simulink model "Vereinfachte_Dehtellersteuerung"  (R2021a)
settings: Solver=ode3  StartTime=0.0  StopTime=10  FixedStep=0.01  RelTol=1e-3
undefined symbols (not defined in the file): A, I, igetr, K, MRK, PHI, Ra, U
settings Model: Creator=Oceaner  LastModifiedBy=Oceaner

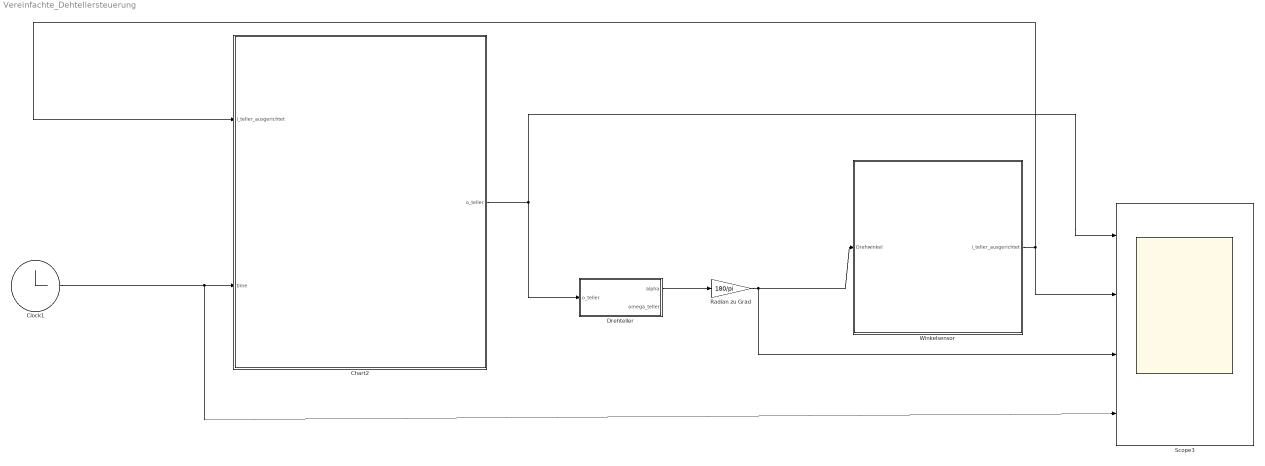
== system Vereinfachte_Dehtellersteuerung ==
  Chart2 : Stateflow chart  TreatAsAtomicUnit=on
  Clock1 : Clock
  Drehteller : Subsystem
  Radian zu Grad : Gain  Gain=180/pi
  Scope3 : Scope  NumInputPorts=4
  Winkelsensor : Stateflow chart  TreatAsAtomicUnit=on
  wires:
  Clock1/1 -> Scope3/4, Chart2/2(time)
  Winkelsensor/1(i_teller_ausgerichtet) -> Chart2/1(i_teller_ausgerichtet), Scope3/2
  Drehteller/1(alpha) -> Radian zu Grad/1
  Chart2/1(o_teller) -> Drehteller/1(o_teller), Scope3/1
  Radian zu Grad/1 -> Scope3/3, Winkelsensor/1(Drehwinkel)

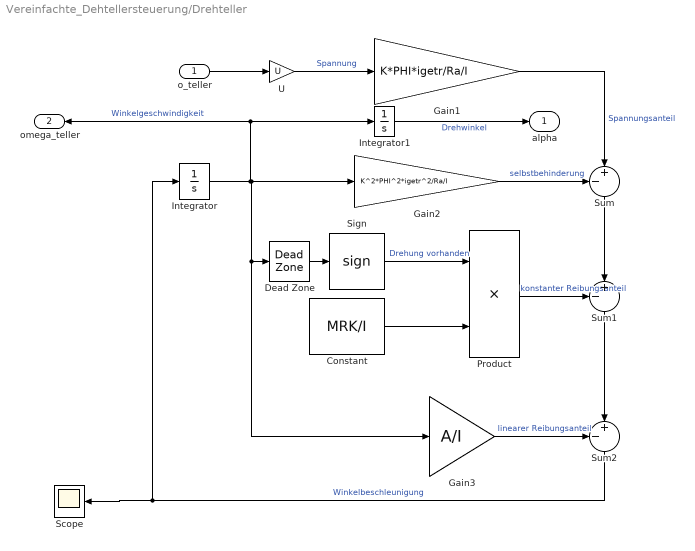
== system Vereinfachte_Dehtellersteuerung/Drehteller ==
  o_teller : Inport
  Constant : Constant  Value=MRK/I
  Dead Zone : DeadZone  SaturateOnIntegerOverflow=on
  Gain1 : Gain  Gain=K*PHI*igetr/Ra/I
  Gain2 : Gain  Gain=K^2*PHI^2*igetr^2/Ra/I
  Gain3 : Gain  Gain=A/I
  Integrator : Integrator
  Integrator1 : Integrator
  Product : Product
  Scope : Scope
  Sign : Signum
  Sum : Sum  Inputs=-+|
  Sum1 : Sum  Inputs=-+|
  Sum2 : Sum  Inputs=-+|
  U : Gain  Gain=U
  alpha : Outport
  omega_teller : Outport  Port=2
  wires:
  U/1 -> Gain1/1  "Spannung"
  Product/1 -> Sum1/1  "konstanter Reibungsanteil"
  Integrator/1 -> Gain2/1, Gain3/1, Dead Zone/1, omega_teller/1, Integrator1/1  "Winkelgeschwindigkeit"
  Gain1/1 -> Sum/2  "Spannungsanteil"
  Sum1/1 -> Sum2/2
  Sum/1 -> Sum1/2
  o_teller/1 -> U/1
  Gain2/1 -> Sum/1  "selbstbehinderung"
  Sign/1 -> Product/1  "Drehung vorhanden"
  Dead Zone/1 -> Sign/1
  Gain3/1 -> Sum2/1  "linearer Reibungsanteil"
  Sum2/1 -> Scope/1, Integrator/1  "Winkelbeschleunigung"
  Constant/1 -> Product/2
  Integrator1/1 -> alpha/1  "Drehwinkel"

== stateflow chart Vereinfachte_Dehtellersteuerung/Chart2 ==
  state pufferstate
  state beginnt
    en:o_teller=1;
  state aus
    en:o_teller=0;
  beginnt -> pufferstate : after(0.5,sec)
  pufferstate -> aus : [i_teller_ausgerichtet==1]
  (default) -> aus
  aus -> beginnt : after(2,sec)
  data: i_teller_ausgerichtet input; time input; o_teller output

== stateflow chart Vereinfachte_Dehtellersteuerung/Winkelsensor ==
  state pause
    en:i_teller_ausgerichtet=1;
  state N
    en:i_teller_ausgerichtet=0;
  pause -> N : [mod(Drehwinkel,90)>2&&mod(Drehwinkel,90)<88]
  N -> pause : [(mod(Drehwinkel,90)>=0&&mod(Drehwinkel,90)<=2)||(mod(Drehwinkel,90)>=88&&mod(Drehwinkel,90)<=90)]
  (default) -> N
  data: Drehwinkel input; i_teller_ausgerichtet output
